simulink library "lib_Serial_PIX"  (R2019b)
settings: Solver=VariableStepAuto  StartTime=0.0  StopTime=10.0  RelTol=1e-3
undefined symbols (not defined in the file or in its folder): HIL_Data, HIL_Sample_Time, serial, Serial_Port, Standard_Devices
libraries: instrumentlib x7, etargetslib x4, aerolibanimutils x2, sldrtlib x2, pixhawk_slib_uORB_RW x1, pixhawk_slib_ADC_serial x1
settings Model: Creator=m.hiepp  LastModifiedBy=guy-m
settings DataIOCC: ReturnWorkspaceOutputs=off
settings DebuggingCC: ArithmeticOperatorsInVariantConditions=warning
settings SFSimCC: CustomCodeUndefinedFunction=UseInterfaceOnly

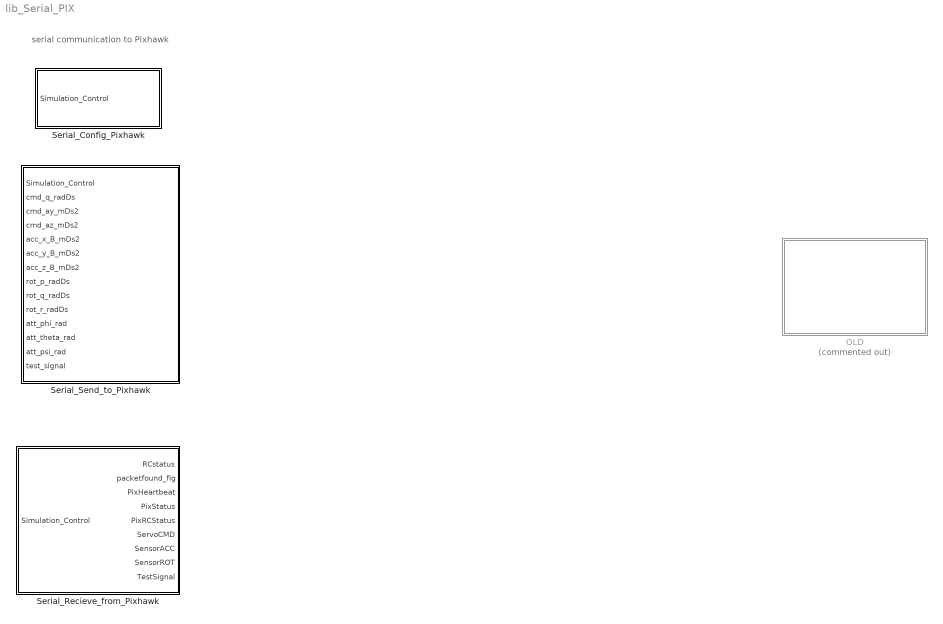
== system lib_Serial_PIX ==
  note: serial communication to Pixhawk
  OLD : Subsystem  Commented=on
  Serial_Config_Pixhawk : Subsystem  mask{Pix=HIL_Data.Serial.Pix}
      mask prompts: Pix "Pix Serial Data"
  Serial_Recieve_from_Pixhawk : Subsystem  mask{Serial=HIL_Data.Serial.Pix}
      mask prompts: Serial "Pix Serial Data"
  Serial_Send_to_Pixhawk : Subsystem  mask{Serial=HIL_Data.Serial.Pix}
      mask prompts: Serial "Pix Serial Data"

== system lib_Serial_PIX/OLD ==
  note: at Pixhawk
  note: at Simulation PC
  Host_Reciever_UART : Subsystem
  Host_Sender_UART : Subsystem
  PIX_Reciever_UART : Subsystem
  PIX_Sender_UART : Subsystem

== system lib_Serial_PIX/Serial_Config_Pixhawk ==
  Simulation_Control : Inport  OutDataTypeStr=Bus: Simulation_Ctrl_Bus
  Bus Selector : BusSelector  OutputSignals=external
  Display : Display
  NOT : Logic  Operator=NOT  IconShape=distinctive  AllPortsSameDT=off  OutDataTypeStr=boolean
  enable_serial_config : Subsystem
  wires:
  Simulation_Control/1 -> Bus Selector/1
  Bus Selector/1 -> NOT/1  "<external>"
  NOT/1 -> Display/1, enable_serial_config/Enable

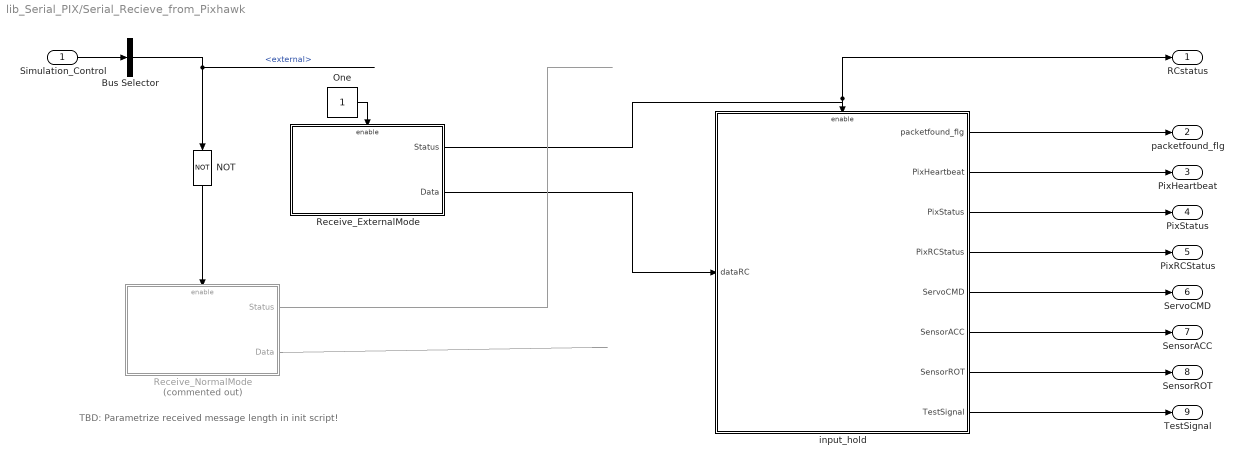
== system lib_Serial_PIX/Serial_Recieve_from_Pixhawk ==
  note: TBD: Parametrize received message length in init script!
  Simulation_Control : Inport  OutDataTypeStr=Bus: Simulation_Ctrl_Bus
  Bus Selector : BusSelector  OutputSignals=external
  NOT : Logic  Operator=NOT  IconShape=distinctive  AllPortsSameDT=off  OutDataTypeStr=boolean
  One : Constant  OutDataTypeStr=Inherit: Inherit via back propagation
  Receive_ExternalMode : Subsystem
  Receive_NormalMode : Subsystem  Commented=on
  input_hold : Subsystem
  RCstatus : Outport  VectorParamsAs1DForOutWhenUnconnected=off
  packetfound_flg : Outport  Port=2  VectorParamsAs1DForOutWhenUnconnected=off
  PixHeartbeat : Outport  Port=3  VectorParamsAs1DForOutWhenUnconnected=off
  PixStatus : Outport  Port=4  VectorParamsAs1DForOutWhenUnconnected=off
  PixRCStatus : Outport  Port=5  VectorParamsAs1DForOutWhenUnconnected=off
  ServoCMD : Outport  Port=6  VectorParamsAs1DForOutWhenUnconnected=off
  SensorACC : Outport  Port=7  VectorParamsAs1DForOutWhenUnconnected=off
  SensorROT : Outport  Port=8  VectorParamsAs1DForOutWhenUnconnected=off
  TestSignal : Outport  Port=9  VectorParamsAs1DForOutWhenUnconnected=off
  wires:
  input_hold/8(TestSignal) -> TestSignal/1
  input_hold/2(PixHeartbeat) -> PixHeartbeat/1
  input_hold/5(ServoCMD) -> ServoCMD/1
  input_hold/6(SensorACC) -> SensorACC/1
  input_hold/7(SensorROT) -> SensorROT/1
  input_hold/1(packetfound_flg) -> packetfound_flg/1
  input_hold/4(PixRCStatus) -> PixRCStatus/1
  input_hold/3(PixStatus) -> PixStatus/1
  Receive_ExternalMode/1(Status) -> RCstatus/1, input_hold/Enable
  Receive_ExternalMode/2(Data) -> input_hold/1(dataRC)
  Simulation_Control/1 -> Bus Selector/1
  Receive_NormalMode/2(Data) -> ?
  NOT/1 -> Receive_NormalMode/Enable
  Bus Selector/1 -> NOT/1  "<external>"
  Receive_NormalMode/1(Status) -> ?
  One/1 -> Receive_ExternalMode/Enable

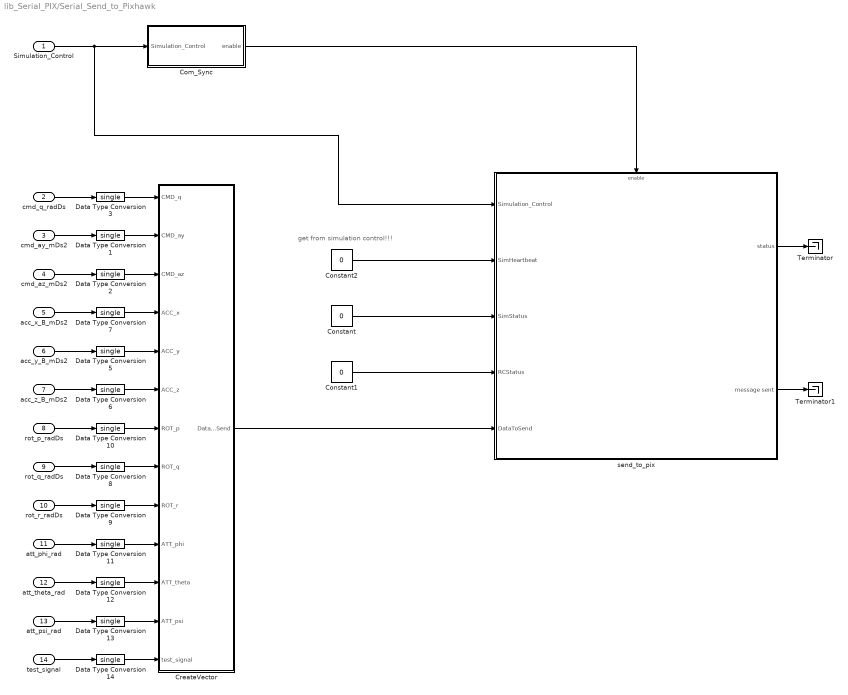
== system lib_Serial_PIX/Serial_Send_to_Pixhawk ==
  note: get from simulation control!!!
  Simulation_Control : Inport  OutDataTypeStr=Bus: Simulation_Ctrl_Bus
  cmd_q_radDs : Inport  Port=2
  cmd_ay_mDs2 : Inport  Port=3
  cmd_az_mDs2 : Inport  Port=4
  acc_x_B_mDs2 : Inport  Port=5
  acc_y_B_mDs2 : Inport  Port=6
  acc_z_B_mDs2 : Inport  Port=7
  rot_p_radDs : Inport  Port=8
  rot_q_radDs : Inport  Port=9
  rot_r_radDs : Inport  Port=10
  att_phi_rad : Inport  Port=11
  att_theta_rad : Inport  Port=12
  att_psi_rad : Inport  Port=13
  test_signal : Inport  Port=14
  Com_Sync : Subsystem
  Constant : Constant  Value=0  OutDataTypeStr=uint8
  Constant1 : Constant  Value=0  OutDataTypeStr=uint8
  Constant2 : Constant  Value=0  OutDataTypeStr=uint16
  CreateVector : MATLAB Function  TreatAsAtomicUnit=on
  Data Type Conversion{1..3,5..14} (13 alike) : DataTypeConversion  OutDataTypeStr=single
  Terminator : Terminator
  Terminator1 : Terminator
  send_to_pix : Subsystem
  wires:
  Data Type Conversion3/1 -> CreateVector/1(CMD_q)
  Data Type Conversion1/1 -> CreateVector/2(CMD_ay)
  Data Type Conversion2/1 -> CreateVector/3(CMD_az)
  Data Type Conversion7/1 -> CreateVector/4(ACC_x)
  Data Type Conversion5/1 -> CreateVector/5(ACC_y)
  Data Type Conversion6/1 -> CreateVector/6(ACC_z)
  Data Type Conversion10/1 -> CreateVector/7(ROT_p)
  Data Type Conversion8/1 -> CreateVector/8(ROT_q)
  Data Type Conversion9/1 -> CreateVector/9(ROT_r)
  cmd_q_radDs/1 -> Data Type Conversion3/1
  cmd_ay_mDs2/1 -> Data Type Conversion1/1
  cmd_az_mDs2/1 -> Data Type Conversion2/1
  acc_x_B_mDs2/1 -> Data Type Conversion7/1
  acc_y_B_mDs2/1 -> Data Type Conversion5/1
  acc_z_B_mDs2/1 -> Data Type Conversion6/1
  rot_p_radDs/1 -> Data Type Conversion10/1
  rot_q_radDs/1 -> Data Type Conversion8/1
  rot_r_radDs/1 -> Data Type Conversion9/1
  Data Type Conversion11/1 -> CreateVector/10(ATT_phi)
  att_phi_rad/1 -> Data Type Conversion11/1
  Constant/1 -> send_to_pix/3(SimStatus)
  send_to_pix/1(status) -> Terminator/1
  send_to_pix/2(message sent) -> Terminator1/1
  Constant1/1 -> send_to_pix/4(RCStatus)
  att_theta_rad/1 -> Data Type Conversion12/1
  att_psi_rad/1 -> Data Type Conversion13/1
  test_signal/1 -> Data Type Conversion14/1
  Data Type Conversion14/1 -> CreateVector/13(test_signal)
  Data Type Conversion13/1 -> CreateVector/12(ATT_psi)
  Data Type Conversion12/1 -> CreateVector/11(ATT_theta)
  Constant2/1 -> send_to_pix/2(SimHeartbeat)
  CreateVector/1(DataToSend) -> send_to_pix/5(DataToSend)
  Com_Sync/1(enable) -> send_to_pix/Enable
  Simulation_Control/1 -> Com_Sync/1(Simulation_Control), send_to_pix/1(Simulation_Control)

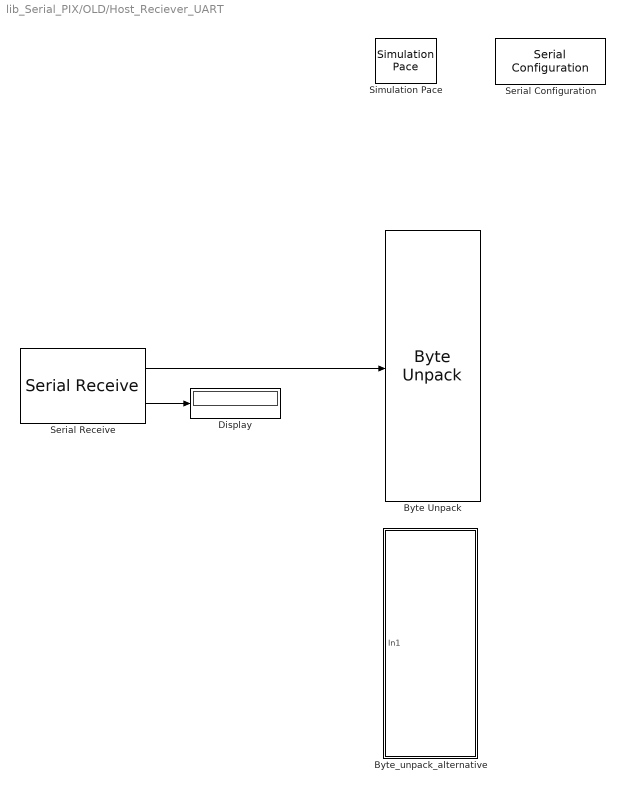
== system lib_Serial_PIX/OLD/Host_Reciever_UART ==
  Byte Unpack : etargetslib/Byte Unpack  dimensions={[1],[1],[1],[1],[1],[1]}  datatypes={'uint8','uint8','single','single','single','uint8'}  byteAlign=1
      settings: SourceProductName=MATLAB Coder
  Byte_unpack_alternative : Subsystem
  Display : Display
  Serial Configuration : instrumentlib/Serial Configuration  Priority=-200000  ComPortMenu=<Please select a port...>  ComPort=COM6  ObjConstructor=serial('COM6');  BaudRate=115200  DataBits=8  Parity=none  StopBits=1  FlowControl=none  Timeout=10  ByteOrder=LittleEndian
  Serial Receive : instrumentlib/Serial Receive  ComPortMenu=<Please select a port...>  ComPort=COM6  ObjConstructor=serial('COM6');  Terminator=<none>  DataSize="[28   1]"  DataType=uint8  EnableBlockingMode=off  ActionDataUnavailable=Output last received value  CustomValue=0  SampleTime=0.005
  Simulation Pace : aerolibanimutils/Simulation Pace  SimulationPace=1  SleepMode=MATLAB Thread  OutputPaceError=off  SampleTime=0.005
  wires:
  Serial Receive/2 -> Display/1
  Serial Receive/1 -> Byte Unpack/1

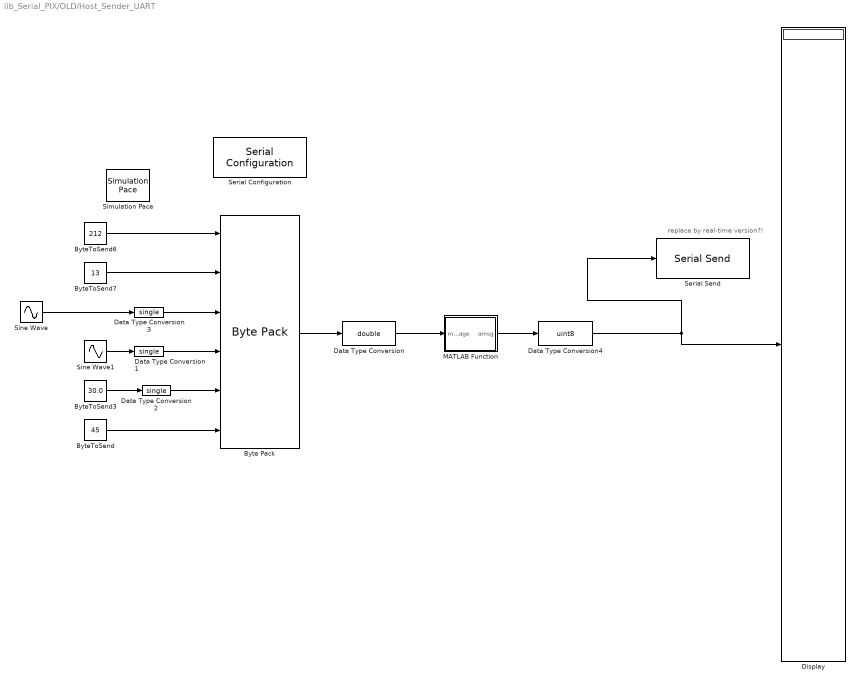
== system lib_Serial_PIX/OLD/Host_Sender_UART ==
  note: replace by real-time version?!
  Byte Pack : etargetslib/Byte Pack  datatypes={'uint8','uint8','single','single','single','uint8'}  byteAlign=1
      settings: SourceProductName=MATLAB Coder
  ByteToSend : Constant  Value=45  OutDataTypeStr=uint8  SampleTime=-1
  ByteToSend3 : Constant  Value=30.0  OutDataTypeStr=single  SampleTime=-1
  ByteToSend6 : Constant  Value=212  OutDataTypeStr=uint8  SampleTime=-1
  ByteToSend7 : Constant  Value=13  OutDataTypeStr=uint8  SampleTime=-1
  Data Type Conversion : DataTypeConversion  OutDataTypeStr=double
  Data Type Conversion1 : DataTypeConversion  OutDataTypeStr=single
  Data Type Conversion2 : DataTypeConversion  OutDataTypeStr=single
  Data Type Conversion3 : DataTypeConversion  OutDataTypeStr=single
  Data Type Conversion4 : DataTypeConversion  OutDataTypeStr=uint8
  Display : Display
  MATLAB Function : MATLAB Function  TreatAsAtomicUnit=on
  Serial Configuration : instrumentlib/Serial Configuration  Priority=-200000  ComPortMenu=<Please select a port...>  ComPort=COM5  ObjConstructor=serial('COM5');  BaudRate=921600  DataBits=8  Parity=none  StopBits=1  FlowControl=none  Timeout=10  ByteOrder=LittleEndian
  Serial Send : instrumentlib/Serial Send  ComPortMenu=<Please select a port...>  ComPort=COM5  ObjConstructor=serial('COM5');  Header=\nn  Terminator=<none>  EnableBlockingMode=off
  Simulation Pace : aerolibanimutils/Simulation Pace  SimulationPace=1  SleepMode=MATLAB Thread  OutputPaceError=off  SampleTime=-1
  Sine Wave : Sin  Amplitude=10  SampleTime=0
  Sine Wave1 : Sin  Amplitude=10  Phase=45*pi/180  SampleTime=0
  wires:
  ByteToSend7/1 -> Byte Pack/2
  Data Type Conversion1/1 -> Byte Pack/4
  Sine Wave1/1 -> Data Type Conversion1/1
  ByteToSend3/1 -> Data Type Conversion2/1
  Data Type Conversion4/1 -> Display/1, Serial Send/1
  Sine Wave/1 -> Data Type Conversion3/1
  Data Type Conversion2/1 -> Byte Pack/5
  ByteToSend6/1 -> Byte Pack/1
  MATLAB Function/1(amsg) -> Data Type Conversion4/1
  Byte Pack/1 -> Data Type Conversion/1
  ByteToSend/1 -> Byte Pack/6
  Data Type Conversion3/1 -> Byte Pack/3
  Data Type Conversion/1 -> MATLAB Function/1(message)

== system lib_Serial_PIX/OLD/PIX_Reciever_UART ==
  note: in the Pixhawk flashed version, the 'Serial Recieve' block
      | is replaced by listening to the respective uORBTopic!!
  Byte Unpack : etargetslib/Byte Unpack  dimensions={[1],[1],[1],[1],[1],[1]}  datatypes={'uint8','uint8','single','single','single','uint8'}  byteAlign=1
      settings: SourceProductName=MATLAB Coder
  uORB Read : pixhawk_slib_uORB_RW/uORB Read // Function-Call Trigger  uORB_Topic_str='sensor_accel'  BusObjVar=Bus: sensor_accel_SL  uORB_Interval=20  AsyncOutput=off  Fcn_call_select=Generate Function Call Signal  TaskName='Task0'  Poll_timeout=100  Ts=-1
  wires:
  uORB Read/1 -> Byte Unpack/1

== system lib_Serial_PIX/OLD/PIX_Sender_UART ==
  Byte Pack : etargetslib/Byte Pack  datatypes={'uint8','uint8','single','single','single','uint8'}  byteAlign=1
      settings: SourceProductName=MATLAB Coder
  Serial Send : pixhawk_slib_ADC_serial/Serial  DeviceName=/dev/ttyACM0  ReadOrWrite=Writing  BaudRateStr=115200  block=off  WriteStatus=on  Terminator=off  Header=off  NumBytesRead=4  TerminatorChar=\n  HeaderData=[ uint8( hex2dec( 'DE' ) ), uint8( hex2dec( 'AD' ) ), uint8( hex2dec( 'C0' ) ), uint8( hex2dec( 'DE' ) ) ]  SimulateUsing=Code generation
  wires:
  Byte Pack/1 -> Serial Send/1

== system lib_Serial_PIX/Serial_Config_Pixhawk/enable_serial_config ==
  Enable : EnablePort
  Serial Configuration : instrumentlib/Serial Configuration  Priority=-200000  ComPortMenu=COM3  ComPort=COM3  ObjConstructor=serial('COM3');  BaudRate=1152000  DataBits=8  Parity=none  StopBits=1  FlowControl=none  Timeout=10  ByteOrder=LittleEndian

== system lib_Serial_PIX/Serial_Recieve_from_Pixhawk/Receive_ExternalMode ==
  note: specify comport and baudrate in block properties!!
  Enable : EnablePort
  AND : Logic  IconShape=distinctive  AllPortsSameDT=off  OutDataTypeStr=boolean
  NOT : Logic  Operator=NOT  IconShape=distinctive  AllPortsSameDT=off  OutDataTypeStr=boolean
  Packet Input : sldrtlib/Packet Input  SampleTime=HIL_Sample_Time  MaxMissedTicks=Serial.Receive.MaxMissedTicks  ShowMissedTicks=off  YieldWhenWaiting=on  DrvName=Standard_Devices/Serial_Port  DrvAddress=1  DrvOptions=[1152000 8 0 0 0 0 0 0]  PacketSize=62  DataTypes='62*uint8'  ShowReady=on  ShowError=on  PacketID=1  ByteOrder=1  ShowTimestamp=off
      settings: AttributesFormatString=Serial Port [1]  SourceProductName=Simulink Desktop Real-Time
  Status : Outport  VectorParamsAs1DForOutWhenUnconnected=off
  Data : Outport  Port=2  VectorParamsAs1DForOutWhenUnconnected=off
  wires:
  Packet Input/3 -> NOT/1
  NOT/1 -> AND/2
  Packet Input/2 -> AND/1
  AND/1 -> Status/1
  Packet Input/1 -> Data/1

== system lib_Serial_PIX/Serial_Recieve_from_Pixhawk/Receive_NormalMode ==
  Enable : EnablePort
  Cast To Boolean : DataTypeConversion  OutDataTypeStr=boolean
  Serial Receive1 : instrumentlib/Serial Receive  ComPortMenu=COM3  ComPort=COM3  ObjConstructor=serial('COM3');  Terminator=<none>  DataSize=62  DataType=uint8  EnableBlockingMode=off  ActionDataUnavailable=Output last received value  CustomValue=0  SampleTime=HIL_Sample_Time
  Status : Outport  VectorParamsAs1DForOutWhenUnconnected=off
  Data : Outport  Port=2  VectorParamsAs1DForOutWhenUnconnected=off
  wires:
  Serial Receive1/1 -> Data/1
  Serial Receive1/2 -> Cast To Boolean/1
  Cast To Boolean/1 -> Status/1

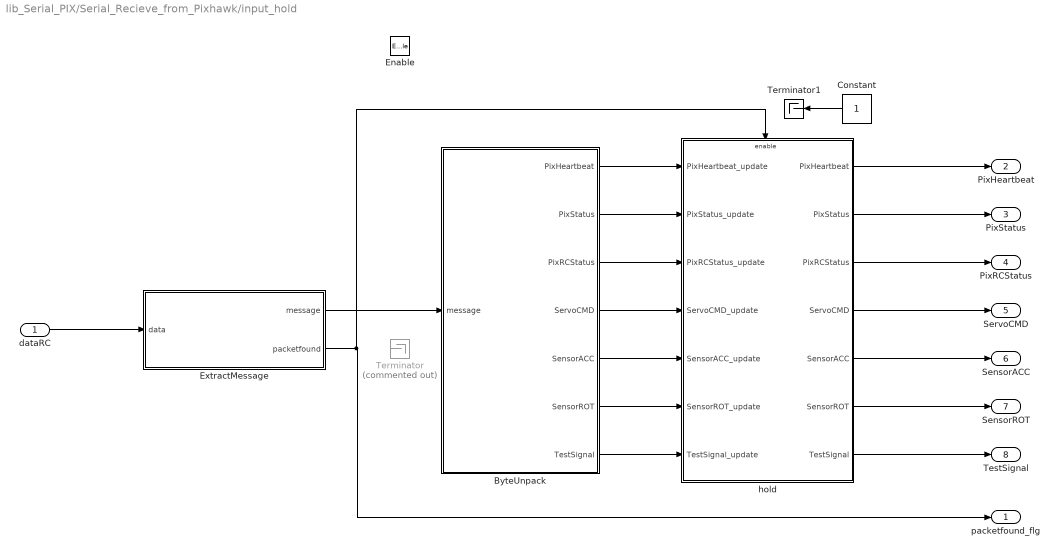
== system lib_Serial_PIX/Serial_Recieve_from_Pixhawk/input_hold ==
  dataRC : Inport
  Enable : EnablePort  PropagateVarSize=During execution
  ByteUnpack : MATLAB Function  TreatAsAtomicUnit=on
  Constant : Constant
  ExtractMessage : MATLAB Function  TreatAsAtomicUnit=on
  Terminator : Terminator  Commented=on
  Terminator1 : Terminator
  hold : Subsystem
  packetfound_flg : Outport  VectorParamsAs1DForOutWhenUnconnected=off
  PixHeartbeat : Outport  Port=2  VectorParamsAs1DForOutWhenUnconnected=off
  PixStatus : Outport  Port=3  VectorParamsAs1DForOutWhenUnconnected=off
  PixRCStatus : Outport  Port=4  VectorParamsAs1DForOutWhenUnconnected=off
  ServoCMD : Outport  Port=5  VectorParamsAs1DForOutWhenUnconnected=off
  SensorACC : Outport  Port=6  VectorParamsAs1DForOutWhenUnconnected=off
  SensorROT : Outport  Port=7  VectorParamsAs1DForOutWhenUnconnected=off
  TestSignal : Outport  Port=8  VectorParamsAs1DForOutWhenUnconnected=off
  wires:
  ExtractMessage/1(message) -> ByteUnpack/1(message)
  dataRC/1 -> ExtractMessage/1(data)
  ExtractMessage/2(packetfound) -> hold/Enable, packetfound_flg/1
  ByteUnpack/1(PixHeartbeat) -> hold/1(PixHeartbeat_update)
  ByteUnpack/2(PixStatus) -> hold/2(PixStatus_update)
  ByteUnpack/3(PixRCStatus) -> hold/3(PixRCStatus_update)
  ByteUnpack/4(ServoCMD) -> hold/4(ServoCMD_update)
  ByteUnpack/5(SensorACC) -> hold/5(SensorACC_update)
  ByteUnpack/6(SensorROT) -> hold/6(SensorROT_update)
  ByteUnpack/7(TestSignal) -> hold/7(TestSignal_update)
  hold/7(TestSignal) -> TestSignal/1
  hold/6(SensorROT) -> SensorROT/1
  hold/5(SensorACC) -> SensorACC/1
  hold/4(ServoCMD) -> ServoCMD/1
  hold/3(PixRCStatus) -> PixRCStatus/1
  hold/2(PixStatus) -> PixStatus/1
  hold/1(PixHeartbeat) -> PixHeartbeat/1
  Constant/1 -> Terminator1/1

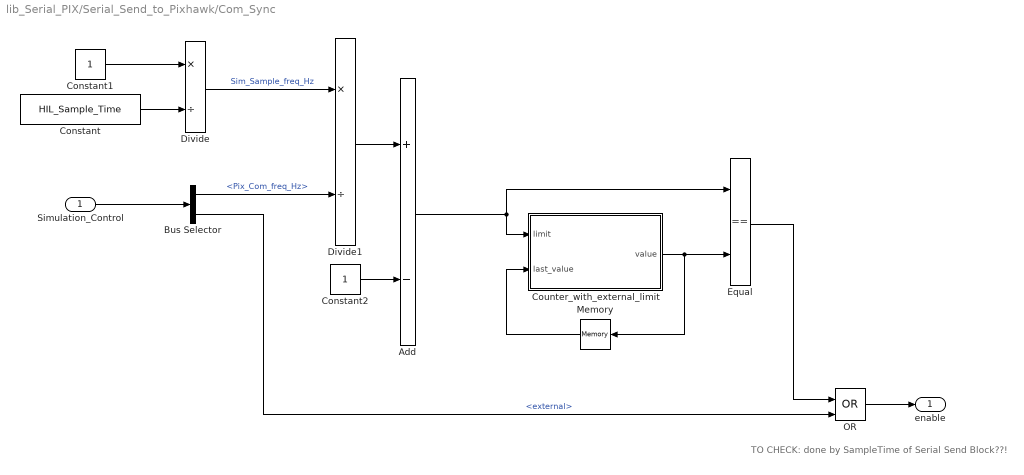
== system lib_Serial_PIX/Serial_Send_to_Pixhawk/Com_Sync ==
  note: TO CHECK: done by SampleTime of Serial Send Block??!
  Simulation_Control : Inport  OutDataTypeStr=Bus: Simulation_Ctrl_Bus
  Add : Sum  Inputs=+-
  Bus Selector : BusSelector  OutputSignals=COM_Ctrl.Pix_Com_freq_Hz,external
  Constant : Constant  Value=HIL_Sample_Time
  Constant1 : Constant
  Constant2 : Constant
  Counter_with_external_limit : MATLAB Function  TreatAsAtomicUnit=on
  Divide : Product  Inputs=*/
  Divide1 : Product  Inputs=*/
  Equal : RelationalOperator  Operator===  OutDataTypeStr=boolean  RndMeth=Simplest
  Memory : Memory  InitialCondition=-1
  OR : Logic  Operator=OR  IconShape=distinctive  AllPortsSameDT=off  OutDataTypeStr=boolean
  enable : Outport  VectorParamsAs1DForOutWhenUnconnected=off
  wires:
  Add/1 -> Counter_with_external_limit/1(limit), Equal/1
  Memory/1 -> Counter_with_external_limit/2(last_value)
  Counter_with_external_limit/1(value) -> Equal/2, Memory/1
  Constant2/1 -> Add/2
  Divide1/1 -> Add/1
  Bus Selector/1 -> Divide1/2  "<Pix_Com_freq_Hz>"
  Divide/1 -> Divide1/1  "Sim_Sample_freq_Hz"
  Constant1/1 -> Divide/1
  Constant/1 -> Divide/2
  Simulation_Control/1 -> Bus Selector/1
  Bus Selector/2 -> OR/2  "<external>"
  Equal/1 -> OR/1
  OR/1 -> enable/1

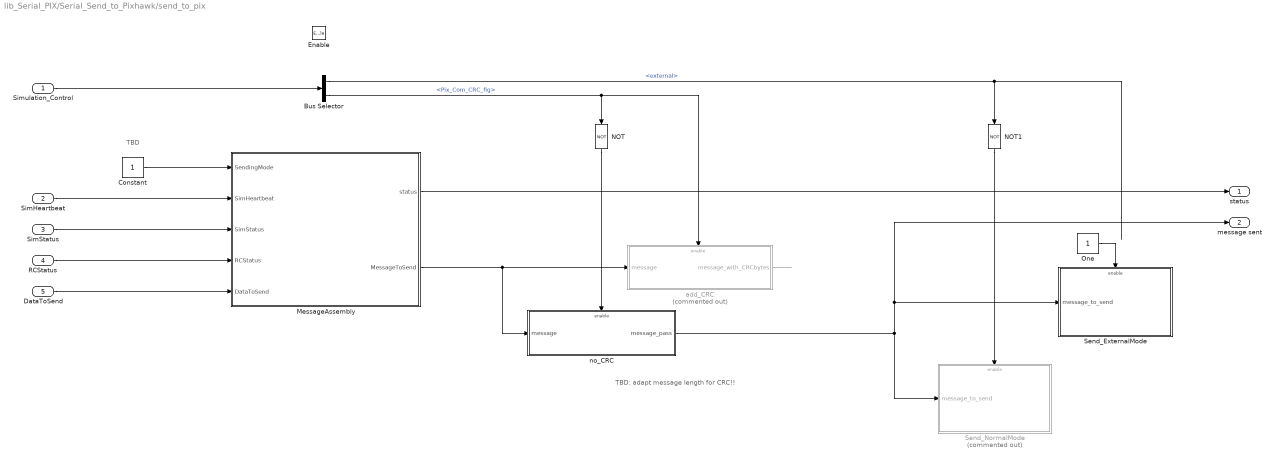
== system lib_Serial_PIX/Serial_Send_to_Pixhawk/send_to_pix ==
  note: TBD
  note: TBD: adapt message length for CRC!!
  Simulation_Control : Inport  OutDataTypeStr=Bus: Simulation_Ctrl_Bus
  SimHeartbeat : Inport  Port=2
  SimStatus : Inport  Port=3
  RCStatus : Inport  Port=4
  DataToSend : Inport  Port=5
  Enable : EnablePort
  Bus Selector : BusSelector  OutputSignals=external,COM_Ctrl.Pix_Com_CRC_flg
  Constant : Constant  OutDataTypeStr=double
  MessageAssembly : MATLAB Function  TreatAsAtomicUnit=on
  NOT : Logic  Operator=NOT  IconShape=distinctive  AllPortsSameDT=off  OutDataTypeStr=boolean
  NOT1 : Logic  Operator=NOT  IconShape=distinctive  AllPortsSameDT=off  OutDataTypeStr=boolean
  One : Constant  OutDataTypeStr=Inherit: Inherit via back propagation
  Send_ExternalMode : Subsystem
  Send_NormalMode : Subsystem  Commented=on
  add_CRC : Subsystem  Commented=on
  no_CRC : Subsystem
  status : Outport  VectorParamsAs1DForOutWhenUnconnected=off
  message sent : Outport  Port=2  VectorParamsAs1DForOutWhenUnconnected=off
  wires:
  Constant/1 -> MessageAssembly/1(SendingMode)
  DataToSend/1 -> MessageAssembly/5(DataToSend)
  RCStatus/1 -> MessageAssembly/4(RCStatus)
  SimStatus/1 -> MessageAssembly/3(SimStatus)
  SimHeartbeat/1 -> MessageAssembly/2(SimHeartbeat)
  MessageAssembly/1(status) -> status/1
  Simulation_Control/1 -> Bus Selector/1
  MessageAssembly/2(MessageToSend) -> no_CRC/1(message), add_CRC/1(message)
  add_CRC/1(message_with_CRCbytes) -> ?
  Bus Selector/1 -> NOT1/1  "<external>"
  Bus Selector/2 -> NOT/1, add_CRC/Enable  "<Pix_Com_CRC_flg>"
  NOT/1 -> no_CRC/Enable
  no_CRC/1(message_pass) -> message sent/1, Send_ExternalMode/1(message_to_send), Send_NormalMode/1(message_to_send)
  NOT1/1 -> Send_NormalMode/Enable
  One/1 -> Send_ExternalMode/Enable

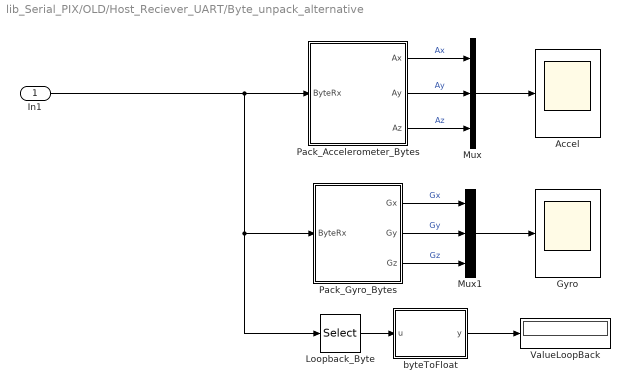
== system lib_Serial_PIX/OLD/Host_Reciever_UART/Byte_unpack_alternative ==
  In1 : Inport
  Accel : Scope
  Gyro : Scope
  Loopback_Byte : Selector  InputPortWidth=28  IndexOptions=Index vector (dialog)  Indices=25:28  OutputSizes=1
  Mux : Mux  Inputs=3
  Mux1 : Mux  Inputs=3
  Pack_Accelerometer_Bytes : Subsystem
  Pack_Gyro_Bytes : Subsystem
  ValueLoopBack : Display
  byteToFloat : MATLAB Function  TreatAsAtomicUnit=on
  wires:
  Mux/1 -> Accel/1
  Pack_Accelerometer_Bytes/2(Ay) -> Mux/2  "Ay"
  byteToFloat/1(y) -> ValueLoopBack/1
  In1/1 -> Pack_Accelerometer_Bytes/1(ByteRx), Loopback_Byte/1, Pack_Gyro_Bytes/1(ByteRx)
  Pack_Gyro_Bytes/2(Gy) -> Mux1/2  "Gy"
  Mux1/1 -> Gyro/1
  Pack_Accelerometer_Bytes/3(Az) -> Mux/3  "Az"
  Loopback_Byte/1 -> byteToFloat/1(u)
  Pack_Gyro_Bytes/3(Gz) -> Mux1/3  "Gz"
  Pack_Gyro_Bytes/1(Gx) -> Mux1/1  "Gx"
  Pack_Accelerometer_Bytes/1(Ax) -> Mux/1  "Ax"

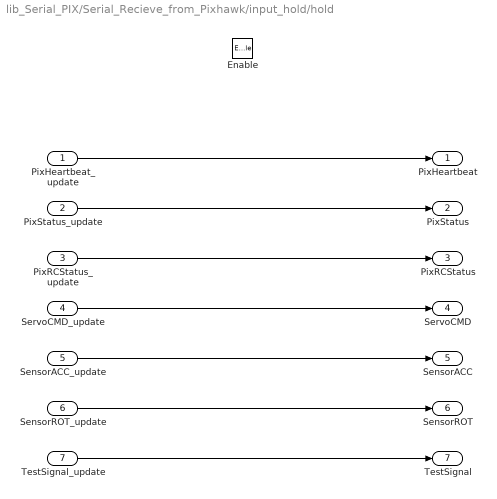
== system lib_Serial_PIX/Serial_Recieve_from_Pixhawk/input_hold/hold ==
  PixHeartbeat_update : Inport
  PixStatus_update : Inport  Port=2
  PixRCStatus_update : Inport  Port=3
  ServoCMD_update : Inport  Port=4
  SensorACC_update : Inport  Port=5
  SensorROT_update : Inport  Port=6
  TestSignal_update : Inport  Port=7
  Enable : EnablePort
  PixHeartbeat : Outport  VectorParamsAs1DForOutWhenUnconnected=off
  PixStatus : Outport  Port=2  VectorParamsAs1DForOutWhenUnconnected=off
  PixRCStatus : Outport  Port=3  VectorParamsAs1DForOutWhenUnconnected=off
  ServoCMD : Outport  Port=4  VectorParamsAs1DForOutWhenUnconnected=off
  SensorACC : Outport  Port=5  VectorParamsAs1DForOutWhenUnconnected=off
  SensorROT : Outport  Port=6  VectorParamsAs1DForOutWhenUnconnected=off
  TestSignal : Outport  Port=7  VectorParamsAs1DForOutWhenUnconnected=off
  wires:
  PixHeartbeat_update/1 -> PixHeartbeat/1
  PixStatus_update/1 -> PixStatus/1
  PixRCStatus_update/1 -> PixRCStatus/1
  ServoCMD_update/1 -> ServoCMD/1
  SensorACC_update/1 -> SensorACC/1
  SensorROT_update/1 -> SensorROT/1
  TestSignal_update/1 -> TestSignal/1

== system lib_Serial_PIX/Serial_Send_to_Pixhawk/send_to_pix/Send_ExternalMode ==
  note: specify comport and baudrate in block porperties!!!
  message_to_send : Inport
  Enable : EnablePort
  Packet Output : sldrtlib/Packet Output  SampleTime=1/HIL_Data.Simulation_Ctrl.Com.Pix.Com_freq_Hz  MaxMissedTicks=Serial.Send.MaxMissedTicks  ShowMissedTicks=off  YieldWhenWaiting=on  DrvName=Standard_Devices/Serial_Port  DrvAddress=1  DrvOptions=[1152000 8 0 0 0 0 0 0]  PacketSize=128  DataTypes='128*uint8'  ShowReady=off  ShowError=on  PacketID=1  ByteOrder=1  InitialValue=[]  FinalValue=[]
      settings: AttributesFormatString=Serial Port [1]  SourceProductName=Simulink Desktop Real-Time
  Terminator : Terminator
  wires:
  message_to_send/1 -> Packet Output/1
  Packet Output/1 -> Terminator/1  "error"

== system lib_Serial_PIX/Serial_Send_to_Pixhawk/send_to_pix/Send_NormalMode ==
  message_to_send : Inport
  Enable : EnablePort
  Serial Send : instrumentlib/Serial Send  ComPortMenu=COM4  ComPort=COM4  ObjConstructor=serial('COM4');  Header=\nn  Terminator=<none>  EnableBlockingMode=off
  wires:
  message_to_send/1 -> Serial Send/1

== system lib_Serial_PIX/Serial_Send_to_Pixhawk/send_to_pix/add_CRC ==
  note: implementation of cyclic redundancy check!!
  message : Inport
  Enable : EnablePort
  Data Type Conversion : DataTypeConversion  OutDataTypeStr=double
  Data Type Conversion4 : DataTypeConversion  OutDataTypeStr=uint8
  MATLAB Function : MATLAB Function  TreatAsAtomicUnit=on
  message_with_CRCbytes : Outport  VectorParamsAs1DForOutWhenUnconnected=off
  wires:
  Data Type Conversion4/1 -> message_with_CRCbytes/1
  MATLAB Function/1(amsg) -> Data Type Conversion4/1
  message/1 -> Data Type Conversion/1
  Data Type Conversion/1 -> MATLAB Function/1(message)

== system lib_Serial_PIX/Serial_Send_to_Pixhawk/send_to_pix/no_CRC ==
  message : Inport
  Enable : EnablePort
  message_pass : Outport  VectorParamsAs1DForOutWhenUnconnected=off
  wires:
  message/1 -> message_pass/1

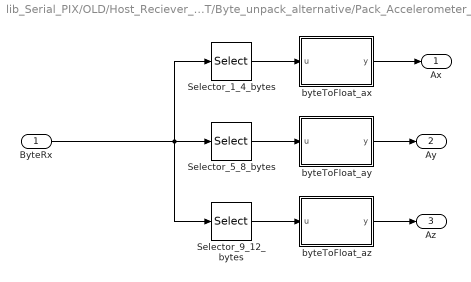
== system lib_Serial_PIX/OLD/Host_Reciever_UART/Byte_unpack_alternative/Pack_Accelerometer_Bytes ==
  ByteRx : Inport
  Selector_1_4_bytes : Selector  InputPortWidth=28  IndexOptions=Index vector (dialog)  Indices=[1:4]  OutputSizes=1
  Selector_5_8_bytes : Selector  InputPortWidth=28  IndexOptions=Index vector (dialog)  Indices=[5 6 7 8]  OutputSizes=1
  Selector_9_12_bytes : Selector  InputPortWidth=28  IndexOptions=Index vector (dialog)  Indices=[9 10 11 12]  OutputSizes=1
  byteToFloat_ax : MATLAB Function  TreatAsAtomicUnit=on
  byteToFloat_ay : MATLAB Function  TreatAsAtomicUnit=on
  byteToFloat_az : MATLAB Function  TreatAsAtomicUnit=on
  Ax : Outport  VectorParamsAs1DForOutWhenUnconnected=off
  Ay : Outport  Port=2  VectorParamsAs1DForOutWhenUnconnected=off
  Az : Outport  Port=3  VectorParamsAs1DForOutWhenUnconnected=off
  wires:
  byteToFloat_az/1(y) -> Az/1
  ByteRx/1 -> Selector_9_12_bytes/1, Selector_1_4_bytes/1, Selector_5_8_bytes/1
  byteToFloat_ax/1(y) -> Ax/1
  Selector_1_4_bytes/1 -> byteToFloat_ax/1(u)
  Selector_9_12_bytes/1 -> byteToFloat_az/1(u)
  Selector_5_8_bytes/1 -> byteToFloat_ay/1(u)
  byteToFloat_ay/1(y) -> Ay/1

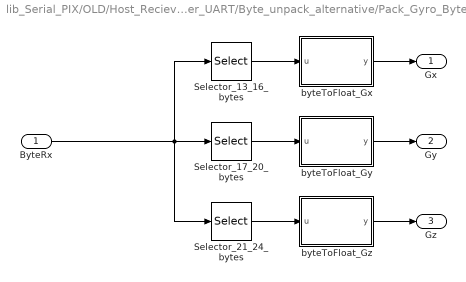
== system lib_Serial_PIX/OLD/Host_Reciever_UART/Byte_unpack_alternative/Pack_Gyro_Bytes ==
  ByteRx : Inport
  Selector_13_16_bytes : Selector  InputPortWidth=28  IndexOptions=Index vector (dialog)  Indices=[13 14 15 16]  OutputSizes=1
  Selector_17_20_bytes : Selector  InputPortWidth=28  IndexOptions=Index vector (dialog)  Indices=[17:20]  OutputSizes=1
  Selector_21_24_bytes : Selector  InputPortWidth=28  IndexOptions=Index vector (dialog)  Indices=[21:24]  OutputSizes=1
  byteToFloat_Gx : MATLAB Function  TreatAsAtomicUnit=on
  byteToFloat_Gy : MATLAB Function  TreatAsAtomicUnit=on
  byteToFloat_Gz : MATLAB Function  TreatAsAtomicUnit=on
  Gx : Outport  VectorParamsAs1DForOutWhenUnconnected=off
  Gy : Outport  Port=2  VectorParamsAs1DForOutWhenUnconnected=off
  Gz : Outport  Port=3  VectorParamsAs1DForOutWhenUnconnected=off
  wires:
  byteToFloat_Gz/1(y) -> Gz/1
  ByteRx/1 -> Selector_21_24_bytes/1, Selector_17_20_bytes/1, Selector_13_16_bytes/1
  byteToFloat_Gx/1(y) -> Gx/1
  Selector_13_16_bytes/1 -> byteToFloat_Gx/1(u)
  Selector_21_24_bytes/1 -> byteToFloat_Gz/1(u)
  Selector_17_20_bytes/1 -> byteToFloat_Gy/1(u)
  byteToFloat_Gy/1(y) -> Gy/1

== matlab function lib_Serial_PIX/OLD/Host_Reciever_UART/Byte_unpack_alternative/Pack_Accelerometer_Bytes/byteToFloat_ax ==
  data: u input; y output
function y = fcn(u)
%#codegen
y = single(0);
y = single(typecast(uint8(u),'single'));
% y = u;

== matlab function lib_Serial_PIX/OLD/Host_Sender_UART/MATLAB Function ==
  data: message input; amsg output
function amsg = crc_Calc(message)
% Appends the crc (Low byte, high byte) to message for modbus
% communication. Message is an array of bytes. Developed for (but not
% limmited to) use with a watlow 96 controller.
amsg = zeros(17,1);
N = length(message);
Crc_ui16LookupTable=[0,4129,8258,12387,16516,20645,24774,28903,33032,37161,41290,45419,49548,...
    53677,57806,61935,4657,528,12915,8786,21173,17044,29431,25302,37689,33560,45947,41818,54205,...
    50076,62463,58334,9314,13379,1056,5121,25830,29895,17572,21637,42346,46411,34088,38153,58862,...
    62927,50604,54669,13907,9842,5649,1584,30423,26358,22165,18100,46939,42874,38681,34616,63455,...
    59390,55197,51132,18628,22757,26758,30887,2112,6241,10242,14371,51660,55789,59790,63919,35144,...
    39273,43274,47403,23285,19156,31415,27286,6769,2640,14899,10770,56317,52188,64447,60318,39801,...
    35672,47931,43802,27814,31879,19684,23749,11298,15363,3168,7233,60846,64911,52716,56781,44330,...
    48395,36200,40265,32407,28342,24277,20212,15891,11826,7761,3696,65439,61374,57309,53244,48923,...
    44858,40793,36728,37256,33193,45514,41451,53516,49453,61774,57711,4224,161,12482,8419,20484,...
    16421,28742,24679,33721,37784,41979,46042,49981,54044,58239,62302,689,4752,8947,13010,16949,...
    21012,25207,29270,46570,42443,38312,34185,62830,58703,54572,50445,13538,9411,5280,1153,29798,...
    25671,21540,17413,42971,47098,34713,38840,59231,63358,50973,55100,9939,14066,1681,5808,26199,...
    30326,17941,22068,55628,51565,63758,59695,39368,35305,47498,43435,22596,18533,30726,26663,6336,...
    2273,14466,10403,52093,56156,60223,64286,35833,39896,43963,48026,19061,23124,27191,31254,2801,6864,...
    10931,14994,64814,60687,56684,52557,48554,44427,40424,36297,31782,27655,23652,19525,15522,11395,...
    7392,3265,61215,65342,53085,57212,44955,49082,36825,40952,28183,32310,20053,24180,11923,16050,3793,7920];

data=[message]; % ~ string '1 2 3 4 5 6 7 8 9'

ui16RetCRC16 = hex2dec('0000');
for I=1:length(data)
    ui8LookupTableIndex = bitxor(data(I),uint8(bitshift(ui16RetCRC16,-8)));
    ui16RetCRC16 = bitxor(Crc_ui16LookupTable(double(ui8LookupTableIndex)+1),mod(bitshift(ui16RetCRC16,8),65536));
end

lowByte = bitand(ui16RetCRC16,hex2dec('ff'));
highByte = bitshift(bitand(ui16RetCRC16,hex2dec('ff00')),-8);

% 
% lowByte = bitand(crc,hex2dec('ff'));
% highByte = bitshift(bitand(crc,hex2dec('ff00')),-8);

amsg(1:N) = message;
amsg(N+1) = lowByte;
amsg(N+2) = highByte;

== matlab function lib_Serial_PIX/OLD/Host_Reciever_UART/Byte_unpack_alternative/Pack_Accelerometer_Bytes/byteToFloat_ay ==
  data: u input; y output
function y = fcn(u)
%#codegen
y = single(0);
y = single(typecast(uint8(u),'single'));
% y = u;

== matlab function lib_Serial_PIX/OLD/Host_Reciever_UART/Byte_unpack_alternative/Pack_Accelerometer_Bytes/byteToFloat_az ==
  data: u input; y output
function y = fcn(u)
%#codegen
y = single(0);
y = single(typecast(uint8(u),'single'));
% y = u;

== matlab function lib_Serial_PIX/OLD/Host_Reciever_UART/Byte_unpack_alternative/Pack_Gyro_Bytes/byteToFloat_Gx ==
  data: u input; y output
function y = fcn(u)
%#codegen
y = single(0);
y = single(typecast(uint8(u),'single'));
% y = u;

== matlab function lib_Serial_PIX/OLD/Host_Reciever_UART/Byte_unpack_alternative/Pack_Gyro_Bytes/byteToFloat_Gy ==
  data: u input; y output
function y = fcn(u)
%#codegen
y = single(0);
y = single(typecast(uint8(u),'single'));
% y = u;

== matlab function lib_Serial_PIX/OLD/Host_Reciever_UART/Byte_unpack_alternative/Pack_Gyro_Bytes/byteToFloat_Gz ==
  data: u input; y output
function y = fcn(u)
%#codegen
y = single(0);
y = single(typecast(uint8(u),'single'));
% y = u;

== matlab function lib_Serial_PIX/OLD/Host_Reciever_UART/Byte_unpack_alternative/byteToFloat ==
  data: u input; y output
function y = fcn(u)
%#codegen
y = single(0);
y = single(typecast(uint8(u),'single'));
% y = u;

== matlab function lib_Serial_PIX/Serial_Send_to_Pixhawk/send_to_pix/add_CRC/MATLAB Function ==
  data: message input double size=[1 32]; amsg output double size=[1 34]
function amsg = crc_Calc(message)
% Appends the crc (Low byte, high byte) to message for modbus
% communication. Message is an array of bytes. Developed for (but not
% limmited to) use with a watlow 96 controller.
N = length(message);
amsg = zeros(N+2,1);
Crc_ui16LookupTable=[0,4129,8258,12387,16516,20645,24774,28903,33032,37161,41290,45419,49548,...
    53677,57806,61935,4657,528,12915,8786,21173,17044,29431,25302,37689,33560,45947,41818,54205,...
    50076,62463,58334,9314,13379,1056,5121,25830,29895,17572,21637,42346,46411,34088,38153,58862,...
    62927,50604,54669,13907,9842,5649,1584,30423,26358,22165,18100,46939,42874,38681,34616,63455,...
    59390,55197,51132,18628,22757,26758,30887,2112,6241,10242,14371,51660,55789,59790,63919,35144,...
    39273,43274,47403,23285,19156,31415,27286,6769,2640,14899,10770,56317,52188,64447,60318,39801,...
    35672,47931,43802,27814,31879,19684,23749,11298,15363,3168,7233,60846,64911,52716,56781,44330,...
    48395,36200,40265,32407,28342,24277,20212,15891,11826,7761,3696,65439,61374,57309,53244,48923,...
    44858,40793,36728,37256,33193,45514,41451,53516,49453,61774,57711,4224,161,12482,8419,20484,...
    16421,28742,24679,33721,37784,41979,46042,49981,54044,58239,62302,689,4752,8947,13010,16949,...
    21012,25207,29270,46570,42443,38312,34185,62830,58703,54572,50445,13538,9411,5280,1153,29798,...
    25671,21540,17413,42971,47098,34713,38840,59231,63358,50973,55100,9939,14066,1681,5808,26199,...
    30326,17941,22068,55628,51565,63758,59695,39368,35305,47498,43435,22596,18533,30726,26663,6336,...
    2273,14466,10403,52093,56156,60223,64286,35833,39896,43963,48026,19061,23124,27191,31254,2801,6864,...
    10931,14994,64814,60687,56684,52557,48554,44427,40424,36297,31782,27655,23652,19525,15522,11395,...
    7392,3265,61215,65342,53085,57212,44955,49082,36825,40952,28183,32310,20053,24180,11923,16050,3793,7920];

data=[message]; % ~ string '1 2 3 4 5 6 7 8 9'

ui16RetCRC16 = hex2dec('0000');
for I=1:length(data)
    ui8LookupTableIndex = bitxor(data(I),uint8(bitshift(ui16RetCRC16,-8)));
    ui16RetCRC16 = bitxor(Crc_ui16LookupTable(double(ui8LookupTableIndex)+1),mod(bitshift(ui16RetCRC16,8),65536));
end

lowByte = bitand(ui16RetCRC16,hex2dec('ff'));
highByte = bitshift(bitand(ui16RetCRC16,hex2dec('ff00')),-8);

% 
% lowByte = bitand(crc,hex2dec('ff'));
% highByte = bitshift(bitand(crc,hex2dec('ff00')),-8);

amsg(1:N) = message;
amsg(N+1) = lowByte;
amsg(N+2) = highByte;

== matlab function lib_Serial_PIX/Serial_Send_to_Pixhawk/CreateVector ==
  data: CMD_q input single size=1; DataToSend output size=[1 13]; CMD_ay input single size=1; CMD_az input single size=1; ACC_x input single size=1; ACC_y input single size=1; ACC_z input single size=1; ROT_p input single size=1; ROT_q input single size=1; ROT_r input single size=1; ATT_phi input single size=1; ATT_theta input single size=1; ATT_psi input single size=1; test_signal input
function DataToSend = CreateVector(CMD_q, CMD_ay, CMD_az, ACC_x, ACC_y, ACC_z, ROT_p, ROT_q, ROT_r, ATT_phi, ATT_theta, ATT_psi, test_signal)
    
    %specify size and type of input and output data in data manager!!
    
    DataToSend = single([CMD_q CMD_ay CMD_az ACC_x ACC_y ACC_z ROT_p ROT_q ROT_r ATT_phi ATT_theta ATT_psi test_signal]);
    
    
end

== matlab function lib_Serial_PIX/Serial_Send_to_Pixhawk/send_to_pix/MessageAssembly ==
  data: SendingMode input double size=1; SimHeartbeat input uint16 size=1; status output double size=1; SimStatus input uint8 size=1; RCStatus input uint8 size=1; DataToSend input single size=[1 13]; MessageToSend output uint8 size=[1 128]
function [status, MessageToSend] = MessageAssembly(SendingMode, SimHeartbeat, SimStatus, RCStatus, DataToSend)
    
    %specify size and type of input and output data in data manager!!
    
    if SendingMode == 1
        
        %DataToSend = DataToSend';
        
        whiteNoise = uint8([0 0 0 0 0]);
        
        package = [typecast(uint16(SimHeartbeat),'uint8') SimStatus RCStatus typecast(single(DataToSend(1)),'uint8') typecast(single(DataToSend(2)),'uint8') typecast(single(DataToSend(3)),'uint8') typecast(single(DataToSend(4)),'uint8') typecast(single(DataToSend(5)),'uint8') typecast(single(DataToSend(6)),'uint8') typecast(single(DataToSend(7)),'uint8') typecast(single(DataToSend(8)),'uint8') typecast(single(DataToSend(9)),'uint8') typecast(single(DataToSend(10)),'uint8') typecast(single(DataToSend(11)),'uint8') typecast(single(DataToSend(12)),'uint8') typecast(single(DataToSend(13)),'uint8')];
        
        headerToSend = uint8([7 7]);
        packetToSend = uint8(package);
        
        MessageToSend = [whiteNoise headerToSend packetToSend headerToSend packetToSend headerToSend whiteNoise];
        
        %fwrite(s,dataToSend);
        %bytes_sent = s.ValuesSent;
        
        status = 0;
    else
        
        MessageToSend = uint8(zeros(1,128));
        status = -1;
        
    end
    
end

== matlab function lib_Serial_PIX/Serial_Recieve_from_Pixhawk/input_hold/ByteUnpack ==
  data: message input uint8 size=[1 48]; PixHeartbeat output uint16 size=1; PixStatus output uint8 size=1; PixRCStatus output uint8 size=1; ServoCMD output single size=4; SensorACC output single size=3; SensorROT output single size=3; TestSignal output single size=1
function [PixHeartbeat,PixStatus,PixRCStatus,ServoCMD,SensorACC,SensorROT,TestSignal] = ByteUnpack(message)
    
    %specify size and type of input and output data in data manager!!
    
    PixHeartbeat = typecast(uint8(message(1:2)),'uint16');
    PixStatus = message(3);
    PixRCStatus = message(4);
    
    
    ServoCMD1 = typecast(uint8(message(5:8)),'single');
    ServoCMD2 = typecast(uint8(message(9:12)),'single');
    ServoCMD3 = typecast(uint8(message(13:16)),'single');
    ServoCMD4 = typecast(uint8(message(17:20)),'single');
    ServoCMD = [ServoCMD1 ServoCMD2 ServoCMD3 ServoCMD4]';
    
    
    SensorACC1 = typecast(uint8(message(21:24)),'single');
    SensorACC2 = typecast(uint8(message(25:28)),'single');
    SensorACC3 = typecast(uint8(message(29:32)),'single');
    SensorACC = [SensorACC1 SensorACC2 SensorACC3]';
    
    
    SensorROT1 = typecast(uint8(message(33:36)),'single');
    SensorROT2 = typecast(uint8(message(37:40)),'single');
    SensorROT3 = typecast(uint8(message(41:44)),'single');
    SensorROT = [SensorROT1 SensorROT2 SensorROT3]';
    
    TestSignal = typecast(uint8(message(45:48)),'single');
    
end

== matlab function lib_Serial_PIX/Serial_Recieve_from_Pixhawk/input_hold/ExtractMessage ==
  data: data input uint8 size=[62 1]; message output uint8 size=[1 48]; packetfound output
function [message,packetfound] = ExtractMessage(data)
    
    %specify size and type of input and output data in data manager!!
    
    data = data';
    expected_message_length = 48; % specify!!
    expected_header = [5 5];      % specify!!
    expected_header_length = length(expected_header);
    expected_packet_length = expected_message_length + expected_header_length;
    
    packet = uint8(zeros(1,expected_message_length));
    packetfound = false;
    
    %% locate packet in data
    
    % First, find possible header start locations; i.e., match the first element in the
    % header.
    start = find(data==expected_header(1));
    
    % Next remove start values that are too close to the end to possibly match
    % the header.
    endVals = start+expected_header_length-1;
    start(endVals>length(data)) = [];
    
    % Next, loop over elements of header, usually much shorter than length of
    % array, to check which possible header start locations are valid still.
    for pattval = 2:expected_header_length
        % check viable locations in array
        locs = expected_header(pattval) == data(start+pattval-1);
        % delete false ones from indices
        start(~locs) = [];
    end
    
    %Packet = Data - Header
    if ~isempty(start)
        for i = 1:(length(start)-1)
            %Verify if the size of data between 2 consecutive header start
            %indices is equal to the expectedPacketSize
            if isequal(start(i+1)-start(i),expected_packet_length)
            
                %Extract the packet by stripping the header from the data
                packet = data(start(i)+expected_header_length:start(i+1)-1);
                if ~isequal(length(packet),(expected_packet_length-expected_header_length))
                    error('ERROR:Wrong packet size');
                end
            
                %Once a valid packet is found, exit the for loop
                packetfound = true;
                break;
            else
                continue
            end
        end
    else
        packetfound = false;
    end
    
    
    
    %% extract message
    
    message = uint8(packet);
    
    
    
    
    
    
end

== matlab function lib_Serial_PIX/Serial_Send_to_Pixhawk/Com_Sync/Counter_with_external_limit ==
  data: limit input; value output; last_value input
function value = Counter(limit,last_value)
    
    if last_value < limit
        value = last_value + 1;
    else
        value = 0;
    end
    
end
